simulink model "CLE3_sim"  (R2019b)
settings: Solver=FixedStepAuto  StartTime=0.0  StopTime=30  FixedStep=0.0001  RelTol=1e-3
values from neighbouring files (symbols this model uses):
  Ahat = [A Gamma*Theta; zeros(size(A)), F]    [cle3.m]
  Bhat = [B;0;0]    [cle3.m]
  Chat = [C,0,0]    [cle3.m]
  Ghat = [G Gd]    [cle3.m]
  Khat = [4;3;2;-2]    [cle3.m]
settings Model: Creator=Tris  LastModifiedBy=Tris

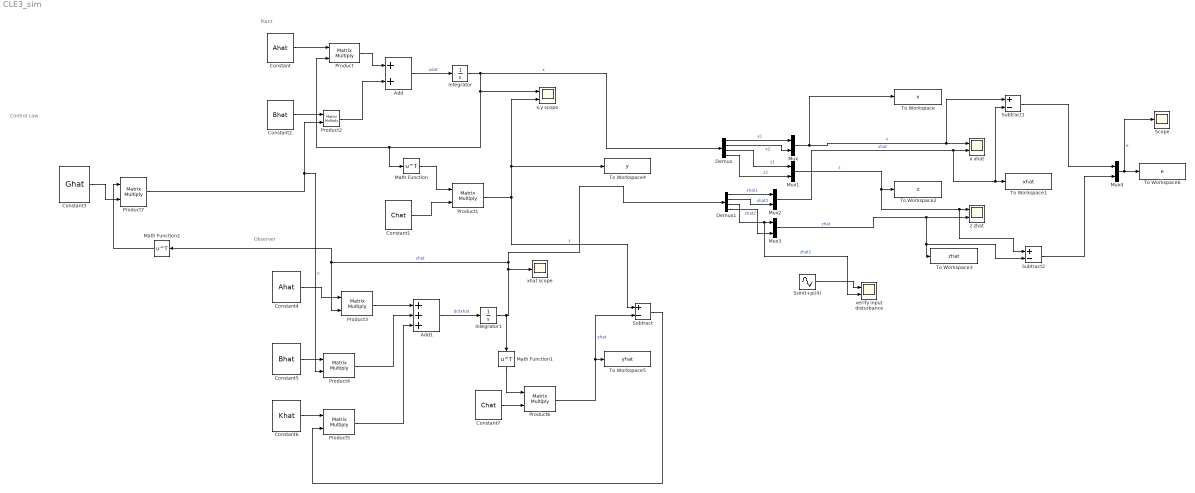
== system CLE3_sim ==
  note: Control Law
  note: Observer
  note: Plant
  5sin(t+pi/4) : Sin  Amplitude=5  Phase=pi/4  SampleTime=0
  Add : Sum
  Add1 : Sum  Inputs=+++
  Constant : Constant  Value=Ahat
  Constant1 : Constant  Value=Chat
  Constant2 : Constant  Value=Bhat
  Constant3 : Constant  Value=Ghat
  Constant4 : Constant  Value=Ahat
  Constant5 : Constant  Value=Bhat
  Constant6 : Constant  Value=Khat
  Constant7 : Constant  Value=Chat
  Demux : Demux
  Demux1 : Demux
  Integrator : Integrator  InitialCondition=5/sqrt(2)
  Integrator1 : Integrator  InitialCondition=1
  Math Function : Math  Operator=transpose  SignedPower=off  SaturateOnIntegerOverflow=on
  Math Function1 : Math  Operator=transpose  SignedPower=off  SaturateOnIntegerOverflow=on
  Math Function2 : Math  Operator=transpose  SignedPower=off  SaturateOnIntegerOverflow=on
  Mux{,1..4} (5 alike) : Mux  Inputs=2
  Product{,1..7} (8 alike) : Product  Multiplication=Matrix(*)
  Scope : Scope
  Subtract : Sum  Inputs=+-
  Subtract1 : Sum  Inputs=+-
  Subtract2 : Sum  Inputs=+-
  To Workspace : ToWorkspace  VariableName=x  SaveFormat=Timeseries  SampleTime=-1
  To Workspace1 : ToWorkspace  VariableName=xhat  SaveFormat=Timeseries  SampleTime=-1
  To Workspace2 : ToWorkspace  VariableName=z  SaveFormat=Timeseries  SampleTime=-1
  To Workspace3 : ToWorkspace  VariableName=zhat  SaveFormat=Timeseries  SampleTime=-1
  To Workspace4 : ToWorkspace  VariableName=y  SaveFormat=Timeseries  SampleTime=-1
  To Workspace5 : ToWorkspace  VariableName=yhat  SaveFormat=Timeseries  SampleTime=-1
  To Workspace6 : ToWorkspace  VariableName=e  SaveFormat=Timeseries  SampleTime=-1
  verify input disturbance : Scope  NumInputPorts=2
  x xhat : Scope  NumInputPorts=2
  x,y scope : Scope  NumInputPorts=2
  xhat scope : Scope
  z zhat : Scope  NumInputPorts=2
  wires:
  Constant/1 -> Product/1
  Product/1 -> Add/1
  Add/1 -> Integrator/1  "xdot"
  Constant2/1 -> Product2/1
  Product2/1 -> Add/2
  Integrator/1 -> Demux/1, x,y scope/1, Math Function/1, Product/2  "x"
  Product1/1 -> Subtract/1, To Workspace4/1, x,y scope/2  "y"
  Constant1/1 -> Product1/2
  Math Function/1 -> Product1/1
  Constant4/1 -> Product3/1
  Product3/1 -> Add1/1
  Constant5/1 -> Product4/1
  Product4/1 -> Add1/2
  Constant6/1 -> Product5/1
  Product5/1 -> Add1/3
  Add1/1 -> Integrator1/1  "dotxhat"
  Integrator1/1 -> Math Function1/1, xhat scope/1, Demux1/1, Product3/2, Math Function2/1  "xhat"
  Constant7/1 -> Product6/2
  Math Function1/1 -> Product6/1
  Product6/1 -> To Workspace5/1, Subtract/2  "yhat"
  Subtract/1 -> Product5/2
  Product7/1 -> Product4/2, Product2/2  "u"
  Constant3/1 -> Product7/2
  Math Function2/1 -> Product7/1
  Demux/1 -> Mux/1  "x1"
  Demux/2 -> Mux/2  "x2"
  5sin(t+pi/4)/1 -> verify input disturbance/1
  Mux/1 -> To Workspace/1, Subtract1/1, x xhat/1  "x"
  Demux/3 -> Mux1/1  "z1"
  Demux/4 -> Mux1/2  "z2"
  Mux1/1 -> To Workspace2/1, Subtract2/1, z zhat/1  "z"
  Demux1/1 -> Mux2/1  "xhat1"
  Demux1/2 -> Mux2/2  "xhat2"
  Mux2/1 -> Subtract1/2, To Workspace1/1, x xhat/2  "xhat"
  Demux1/3 -> verify input disturbance/2, Mux3/1  "zhat1"
  Demux1/4 -> Mux3/2  "zhat2"
  Mux3/1 -> Subtract2/2, To Workspace3/1, z zhat/2  "zhat"
  Subtract1/1 -> Mux4/1
  Subtract2/1 -> Mux4/2
  Mux4/1 -> Scope/1, To Workspace6/1  "e"
